simulink model "Pitch_compute"  (R2019b)
settings: Solver=FixedStepAuto  StartTime=0.0  StopTime=inf  RelTol=1e-3  EnableMultiTasking=on
libraries: arduinolib x2, simulink x1
settings Model: SILPILModeSetting=veronly  ExtModeTrigDuration=2  Creator=Anas  LastModifiedBy=Anas
settings OptimizationCC: EnhancedBackFolding=on  PassReuseOutputArgsAs=Individual arguments  ZeroExternalMemoryAtStartup=off  ZeroInternalMemoryAtStartup=off  MaxStackSize=64  OptimizeBlockOrder=speed  DifferentSizesBufferReuse=on  OptimizationCustomize=off  EfficientTunableParamExpr=on
settings DebuggingCC: ParameterTunabilityLossMsg=error
settings HardwareCC: ProdBitPerInt=16  ProdBitPerPointer=16  ProdBitPerSizeT=16  ProdBitPerPtrDiffT=16  ProdLargestAtomicFloat=None  ProdWordSize=8  ProdHWDeviceType=Atmel->AVR
settings SFSimCC: MATLABDynamicMemAlloc=off
settings RTWCC: SystemTargetFile=ert.tlc  HardwareBoard=Arduino Uno  TLCOptions=-aInlineSetEventsForThisBaseRateFcn=TLC_FALSE -aSuppressMultiTaskScheduler=TLC_FALSE -aRateBasedStepFcn=1  TemplateMakefile=ert_default_tmf  GenerateReport=on  Toolchain=Arduino AVR  BuildConfiguration=Faster Runs  IncludeHyperlinkInReport=on  LaunchReport=on  GenerateTraceInfo=on  GenerateTraceReport=on  GenerateTraceReportSl=on  GenerateTraceReportSf=on  GenerateTraceReportEml=on
settings CodeAppCC: ForceParamTrailComments=on  IgnoreCustomStorageClasses=off  OperatorAnnotations=on  SimulinkDataObjDesc=on  SFDataObjDesc=on  InsertBlockDesc=on
settings ERTTargetCC: SupportContinuousTime=on  SupportVariableSizeSignals=on  ExtModeStaticAllocSize=250

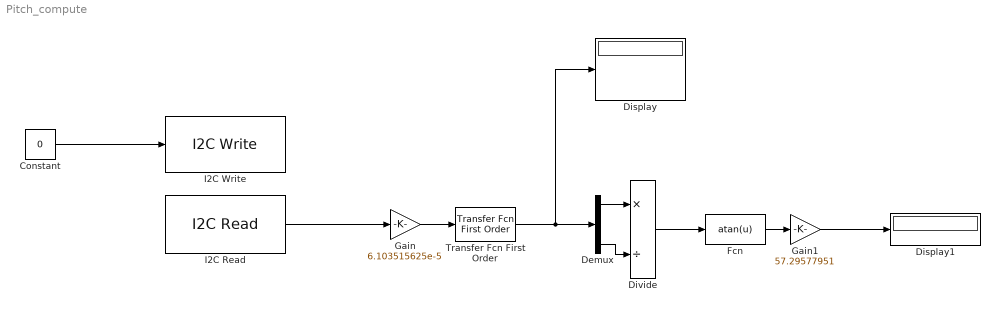
== system Pitch_compute ==
  Constant : Constant  Value=0
  Demux : Demux  Outputs=3
  Display : Display
  Display1 : Display
  Divide : Product  Inputs=*/  OutDataTypeStr=single
  Fcn : Fcn  Expr=atan(u)
  Gain : Gain  Gain=6.103515625e-5
  Gain1 : Gain  Gain=57.29577951
  I2C Read : arduinolib/I2C Read  I2CModule=0  Mode=Master  SlaveAddress=104  SlaveByteOrder=BigEndian  Direction=Receiver  RegisterAddressMode=on  RegisterAddress=0x3B  SlaveDataType=int16  DataLength=3  NoAck=off  RepeatedStart=off  OutputStatus=off  blockPlatform=ARDUINO  SampleTime=-1
      settings: SourceProductName=Simulink Support Package for Arduino Hardware  SourceProductBaseCode=ARDUINO
  I2C Write : arduinolib/I2C Write  I2CModule=0  Mode=Master  SlaveAddress=104  SlaveByteOrder=BigEndian  Direction=Transmitter  RegisterAddressMode=on  RegisterAddress=107  SlaveDataType=uint8  DataLength=1  NoAck=off  RepeatedStart=off  OutputStatus=off  blockPlatform=ARDUINO
      settings: SourceProductName=Simulink Support Package for Arduino Hardware  SourceProductBaseCode=ARDUINO
  Transfer Fcn First Order : simulink/Discrete/Transfer Fcn First Order  PoleZ=0.5  ICPrevOutput=0.0  RndMeth=Nearest  DoSatur=off
      settings: SourceProductName=Simulink
  wires:
  Constant/1 -> I2C Write/1
  I2C Read/1 -> Gain/1
  Gain/1 -> Transfer Fcn First Order/1
  Transfer Fcn First Order/1 -> Demux/1, Display/1
  Demux/1 -> Divide/1
  Demux/3 -> Divide/2
  Divide/1 -> Fcn/1
  Fcn/1 -> Gain1/1
  Gain1/1 -> Display1/1
